simulink model "autolayoutdemo_generated"  (Simulink 7.8)
settings: Solver=ode45  StartTime=0.0  StopTime=10.0  RelTol=1e-3
settings Model: Creator=Ben  LastModifiedBy=Ben

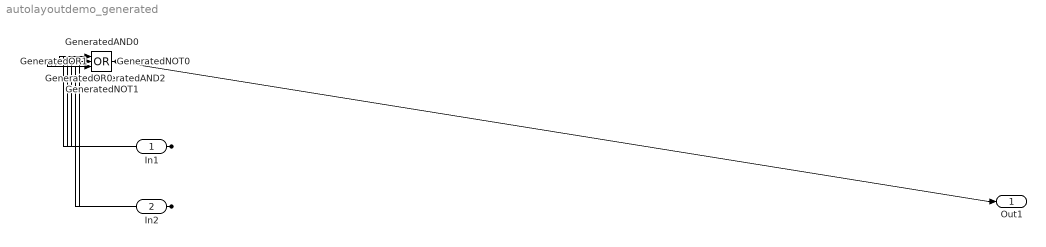
== system autolayoutdemo_generated ==
  In1 : Inport
  In2 : Inport  Port=2
  GeneratedAND0 : Logic
  GeneratedAND2 : Logic  Inputs=3
  GeneratedNOT0 : Logic  Operator=NOT
  GeneratedNOT1 : Logic  Operator=NOT
  GeneratedOR0 : Logic  Operator=OR
  GeneratedOR1 : Logic  Operator=OR
  Out1 : Outport
  wires:
  In2/1 -> GeneratedNOT0/1, GeneratedAND0/2
  In1/1 -> GeneratedNOT1/1, GeneratedOR1/1, GeneratedAND2/1
  GeneratedNOT1/1 -> GeneratedAND0/1
  GeneratedNOT0/1 -> GeneratedOR0/1, GeneratedOR1/2
  GeneratedAND0/1 -> GeneratedOR0/2
  GeneratedOR0/1 -> GeneratedAND2/2
  GeneratedOR1/1 -> GeneratedAND2/3
  GeneratedAND2/1 -> Out1/1
